simulink model "SplPolyInt"  (Simulink 7.9)
settings: Solver=FixedStepDiscrete  StartTime=0.0  StopTime=1023  RelTol=1e-3
libraries: arithm_alteradspbuilder x19, store_alteradspbuilder x13, bus_alteradspbuilder x8, dspsigops x1
Description:
  | 10 разрядный сплайн-интерполятор.
  | Повышение частоты дискретизации в 4 раза.
  | Использует кубический эрмитов сплайн.
settings Model: Creator="Igor Shelevitsky   sheleviv@mail.ru"  ModifiedByFormat=igors  LastModifiedBy=igors
settings OptimizationCC: BooleanDataType=off
settings DebuggingCC: SaveWithParameterizedLinksMsg=none  SignalResolutionControl=TryResolveAllWithWarning  SolverPrmCheckMsg=none  MultiTaskDSMMsg=warning  MultiTaskCondExecSysMsg=none  StrictBusMsg=None
settings HardwareCC: TargetUnknown=on
settings RTWCC: IncludeERTFirstTime=on
settings GRTTargetCC: CombineOutputUpdateFcns=off  GRTInterface=on

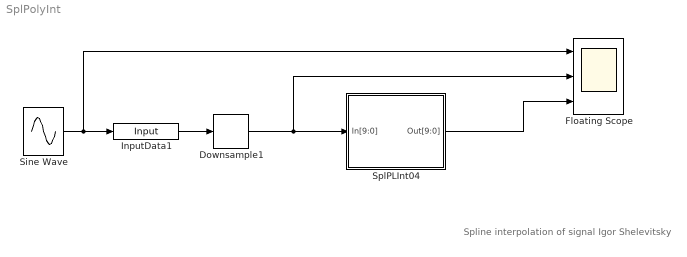
== system SplPolyInt ==
  note: Spline interpolation of signal
      |  Igor Shelevitsky
  Downsample1 : dspsigops/Downsample  N=2  phase=0  InputProcessing=Columns as channels (frame based)  RateOptions=Enforce single-rate processing  smode=Allow multirate  fmode=Maintain input frame size  ic=0
  Floating Scope : Scope  NumInputPorts=3
      settings: TimeRange=128  YMin=-1000~-1000~-1200  YMax=1000~1000~1200
  InputData1 : bus_alteradspbuilder/Input  Description=Sign Binary Fractionnal  sgn=Signed Integer  nodetype=Input Port  bwl=10  bwr=8  sat=off  rnd=off  bp=off  mask_cst=0  LocPin=any  cst=0  modulename=InputData1  ppat=D:\MATLAB6p1\work\DSPBuilder_SPLIc_altera  nSgCpl=0
  Sine Wave : Sin  Amplitude=512  Frequency=0.1  SampleTime=1
  SplPLInt04 : Subsystem  AncestorBlock=ALTELINK/AltLab/HDL SubSystem
      mask Type: SubSystem AlteraBlockSet
  wires:
  Sine Wave/1 -> InputData1/1, Floating Scope/1
  InputData1/1 -> Downsample1/1
  Downsample1/1 -> Floating Scope/2, SplPLInt04/1(In[9:0])
  SplPLInt04/1(Out[9:0]) -> Floating Scope/3

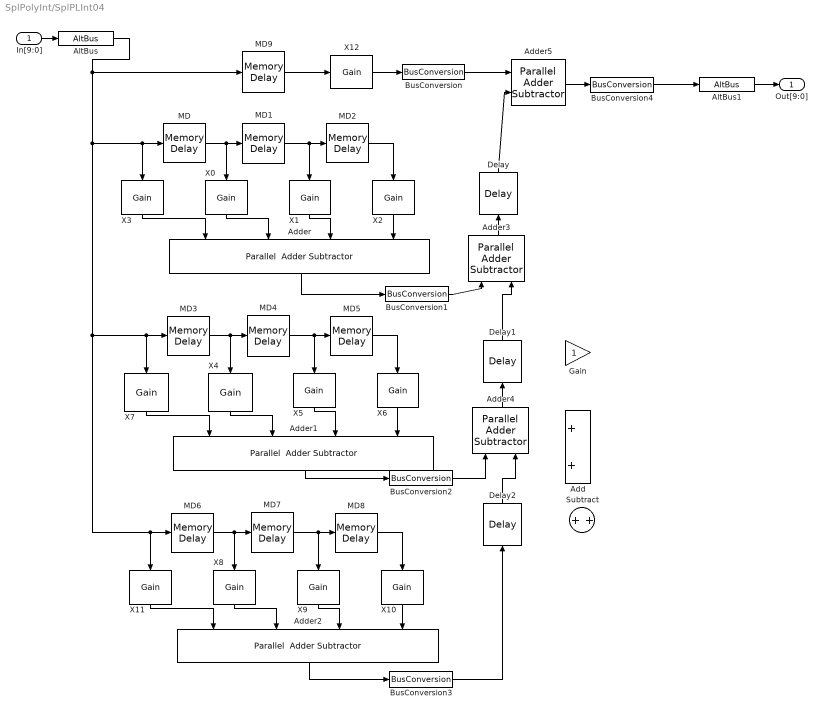
== system SplPolyInt/SplPLInt04 ==
  In[9:0] : Inport
  Add : Sum
  Adder : arithm_alteradspbuilder/Parallel  Adder Subtractor  Inputs=4  direction=++++  pipeline=off  clken=off  MaskValue=1
  Adder1 : arithm_alteradspbuilder/Parallel  Adder Subtractor  Inputs=4  direction=++++  pipeline=off  clken=off  MaskValue=1
  Adder2 : arithm_alteradspbuilder/Parallel  Adder Subtractor  Inputs=4  direction=++++  pipeline=off  clken=off  MaskValue=1
  Adder3 : arithm_alteradspbuilder/Parallel  Adder Subtractor  Inputs=2  direction=++  pipeline=off  clken=off  MaskValue=1
  Adder4 : arithm_alteradspbuilder/Parallel  Adder Subtractor  Inputs=2  direction=++  pipeline=off  clken=off  MaskValue=1
  Adder5 : arithm_alteradspbuilder/Parallel  Adder Subtractor  Inputs=2  direction=++  pipeline=off  clken=off  MaskValue=1
  AltBus : bus_alteradspbuilder/AltBus  Description=Sign Binary Fractionnal  sgn=Signed Integer  nodetype=Input Port  bwl=10  bwr=8  sat=off  rnd=off  bp=off  mask_cst=0  LocPin=any  cst=0  modulename=AltBus  nSgCpl=0
  AltBus1 : bus_alteradspbuilder/AltBus  Description=Sign Binary Fractionnal  sgn=Signed Integer  nodetype=Output Port  bwl=10  bwr=8  sat=off  rnd=off  bp=off  mask_cst=0  LocPin=any  cst=0  modulename=AltBus1  nSgCpl=0
  BusConversion{,1..3} (4 alike) : bus_alteradspbuilder/BusConversion  Inputs=Signed Integer  bwl=23  bwr=8  Outputs=Signed Integer  obwl=14  obwr=0  msb=22  lsb=9  rnd=off  sat=off
  BusConversion4 : bus_alteradspbuilder/BusConversion  Inputs=Signed Integer  bwl=15  bwr=8  Outputs=Signed Integer  obwl=10  obwr=0  msb=14  lsb=5  rnd=off  sat=off
  Delay : store_alteradspbuilder/Delay  depth=1  clken=off  MaskValue=1
  Delay1 : store_alteradspbuilder/Delay  depth=1  clken=off  MaskValue=1
  Delay2 : store_alteradspbuilder/Delay  depth=1  clken=off  MaskValue=1
  Gain : Gain
  MD{,1..9} (10 alike) : store_alteradspbuilder/Memory Delay  bwaddr=1  depth=4  cst=off  clken=off  eab=on  vDepthAltr=4
  Subtract : Sum
  X0 : arithm_alteradspbuilder/Gain  vgain=928  BusType=Signed Integer  bwl=14  bwr=0  pipeline=0  lpm=off  clken=off  gain=928  MaskValue=1
  X1 : arithm_alteradspbuilder/Gain  vgain=3552  BusType=Signed Integer  bwl=14  bwr=0  pipeline=0  lpm=off  clken=off  gain=3552  MaskValue=1
  X10 : arithm_alteradspbuilder/Gain  vgain=-96  BusType=Signed Integer  bwl=14  bwr=0  pipeline=0  lpm=off  clken=off  gain=-96  MaskValue=1
  X11 : arithm_alteradspbuilder/Gain  vgain=-288  BusType=Signed Integer  bwl=14  bwr=0  pipeline=0  lpm=off  clken=off  gain=-288  MaskValue=1
  X12 : arithm_alteradspbuilder/Gain  vgain=4096  BusType=Signed Integer  bwl=14  bwr=0  pipeline=0  lpm=off  clken=off  gain=4096  MaskValue=1
  X2 : arithm_alteradspbuilder/Gain  vgain=-288  BusType=Signed Integer  bwl=14  bwr=0  pipeline=0  lpm=off  clken=off  gain=-288  MaskValue=1
  X3 : arithm_alteradspbuilder/Gain  vgain=-96  BusType=Signed Integer  bwl=14  bwr=0  pipeline=0  lpm=off  clken=off  gain=-96  MaskValue=1
  X4 : arithm_alteradspbuilder/Gain  vgain=2304  BusType=Signed Integer  bwl=14  bwr=0  pipeline=0  lpm=off  clken=off  gain=2304  MaskValue=1
  X5 : arithm_alteradspbuilder/Gain  vgain=2304  BusType=Signed Integer  bwl=14  bwr=0  pipeline=0  lpm=off  clken=off  gain=2304  MaskValue=1
  X6 : arithm_alteradspbuilder/Gain  vgain=-256  BusType=Signed Integer  bwl=14  bwr=0  pipeline=0  lpm=off  clken=off  gain=-256  MaskValue=1
  X7 : arithm_alteradspbuilder/Gain  vgain=-256  BusType=Signed Integer  bwl=14  bwr=0  pipeline=0  lpm=off  clken=off  gain=-256  MaskValue=1
  X8 : arithm_alteradspbuilder/Gain  vgain=3552  BusType=Signed Integer  bwl=14  bwr=0  pipeline=0  lpm=off  clken=off  gain=3552  MaskValue=1
  X9 : arithm_alteradspbuilder/Gain  vgain=928  BusType=Signed Integer  bwl=14  bwr=0  pipeline=0  lpm=off  clken=off  gain=928  MaskValue=1
  Out[9:0] : Outport
  wires:
  AltBus1/1 -> Out[9:0]/1
  In[9:0]/1 -> AltBus/1
  AltBus/1 -> MD/1, X3/1, MD3/1, X7/1, MD6/1, X11/1, MD9/1
  MD/1 -> X0/1, MD1/1
  X2/1 -> Adder/4
  X1/1 -> Adder/3
  X0/1 -> Adder/2
  X3/1 -> Adder/1
  MD1/1 -> MD2/1, X1/1
  MD2/1 -> X2/1
  MD3/1 -> X4/1, MD4/1
  X6/1 -> Adder1/4
  X5/1 -> Adder1/3
  X4/1 -> Adder1/2
  X7/1 -> Adder1/1
  MD4/1 -> MD5/1, X5/1
  MD5/1 -> X6/1
  MD6/1 -> X8/1, MD7/1
  X10/1 -> Adder2/4
  X9/1 -> Adder2/3
  X8/1 -> Adder2/2
  X11/1 -> Adder2/1
  MD7/1 -> MD8/1, X9/1
  MD8/1 -> X10/1
  Adder3/1 -> Delay/1
  Adder4/1 -> Delay1/1
  Delay1/1 -> Adder3/2
  Delay2/1 -> Adder4/2
  MD9/1 -> X12/1
  Delay/1 -> Adder5/2
  X12/1 -> BusConversion/1
  BusConversion/1 -> Adder5/1
  Adder/1 -> BusConversion1/1
  BusConversion1/1 -> Adder3/1
  BusConversion2/1 -> Adder4/1
  Adder1/1 -> BusConversion2/1
  Adder2/1 -> BusConversion3/1
  BusConversion3/1 -> Delay2/1
  Adder5/1 -> BusConversion4/1
  BusConversion4/1 -> AltBus1/1
